simulink model "FA_18_Model_2016b"  (R2018a)
settings: Solver=ode45  StartTime=0.0  StopTime=700  FixedStep=0.1  MaxStep=0.1  RelTol=1e-3
PreLoadFcn:
  | load('FA_18_Parameters.mat')
undefined symbols (not defined in the file or in its folder): Earth, WGS84
libraries: aerolibfltsims x1, aerolibtransform2 x1, aerolibconvert2 x1
settings Model: Creator=User  LastModifiedBy=User
settings CodeAppCC: StateflowObjectComments=on

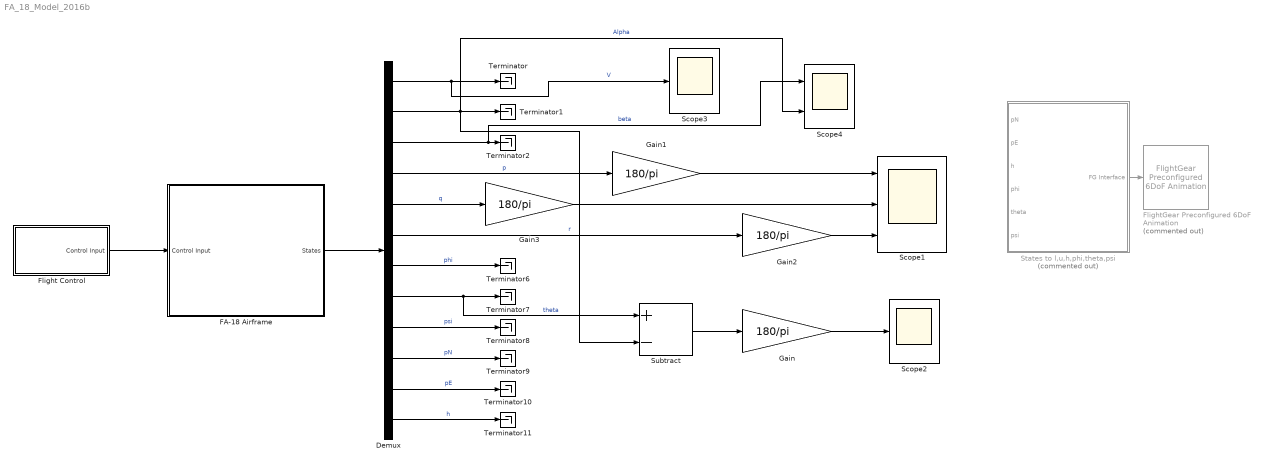
== system FA_18_Model_2016b ==
  Demux : Demux  Outputs=12
  FA-18 Airframe : Subsystem
  Flight Control : Subsystem
  FlightGear Preconfigured 6DoF Animation : aerolibfltsims/FlightGear Preconfigured 6DoF Animation  Commented=on  xFlightGearVersion=v2017.3  DestinationIpAddress=127.0.0.1  DestinationPort=5502  SampleTime=1/30
      settings: SourceProductName=Aerospace Blockset
  Gain{,1..3} (4 alike) : Gain  Gain=180/pi
  Scope1 : Scope  NumInputPorts=3
  Scope2 : Scope
  Scope3 : Scope
  Scope4 : Scope  NumInputPorts=2
  States to l,u,h,phi,theta,psi : Subsystem  Commented=on
  Subtract : Sum  Inputs=+-
  Terminator{,1..2,6..11} (9 alike) : Terminator
  wires:
  States to l,u,h,phi,theta,psi/1(FG Interface) -> FlightGear Preconfigured 6DoF Animation/1
  Flight Control/1(Control Input) -> FA-18 Airframe/1(Control Input)
  Demux/3 -> Scope4/1, Terminator2/1  "beta"
  Demux/2 -> Terminator1/1, Subtract/2, Scope4/2  "Alpha"
  Demux/8 -> Terminator7/1, Subtract/1  "theta"
  Demux/1 -> Scope3/1, Terminator/1  "V"
  Demux/7 -> Terminator6/1  "phi"
  Demux/4 -> Gain1/1  "p"
  Demux/10 -> Terminator9/1  "pN"
  Demux/9 -> Terminator8/1  "psi"
  FA-18 Airframe/1(States) -> Demux/1
  Demux/11 -> Terminator10/1  "pE"
  Demux/6 -> Gain2/1  "r"
  Demux/12 -> Terminator11/1  "h"
  Subtract/1 -> Gain/1
  Gain/1 -> Scope2/1
  Demux/5 -> Gain3/1  "q"
  Gain1/1 -> Scope1/1
  Gain2/1 -> Scope1/3
  Gain3/1 -> Scope1/2

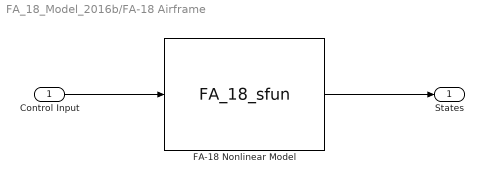
== system FA_18_Model_2016b/FA-18 Airframe ==
  Control Input : Inport
  FA-18 Nonlinear Model : S-Function  FunctionName=FA_18_sfun  Parameters=x0  SFunctionDeploymentMode=off  EnableBusSupport=off
  States : Outport
  wires:
  Control Input/1 -> FA-18 Nonlinear Model/1
  FA-18 Nonlinear Model/1 -> States/1

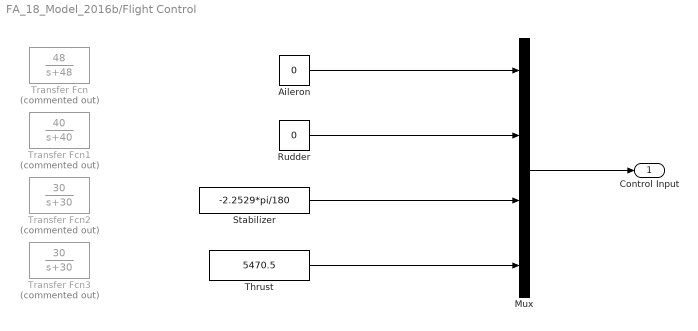
== system FA_18_Model_2016b/Flight Control ==
  Aileron : Constant  Value=0
  Mux : Mux
  Rudder : Constant  Value=0
  Stabilizer : Constant  Value=-2.2529*pi/180
  Thrust : Constant  Value=5470.5
  Transfer Fcn : TransferFcn  Commented=on  Numerator=48  Denominator=[1 48]
  Transfer Fcn1 : TransferFcn  Commented=on  Numerator=[40]  Denominator=[1 40]
  Transfer Fcn2 : TransferFcn  Commented=on  Numerator=[30]  Denominator=[1 30]
  Transfer Fcn3 : TransferFcn  Commented=on  Numerator=[30]  Denominator=[1 30]
  Control Input : Outport
  wires:
  Rudder/1 -> Mux/2
  Thrust/1 -> Mux/4
  Mux/1 -> Control Input/1
  Stabilizer/1 -> Mux/3
  Aileron/1 -> Mux/1

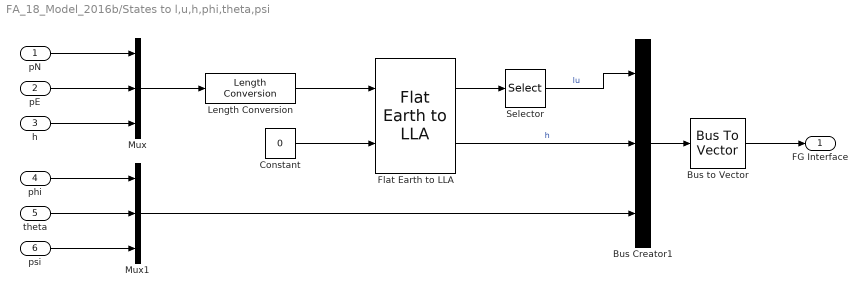
== system FA_18_Model_2016b/States to l,u,h,phi,theta,psi ==
  pN : Inport
  pE : Inport  Port=2
  h : Inport  Port=3
  phi : Inport  Port=4
  theta : Inport  Port=5
  psi : Inport  Port=6
  Bus Creator1 : BusCreator  Inputs=3
  Bus to Vector : BusToVector
  Constant : Constant  Value=0
  Flat Earth to LLA : aerolibtransform2/Flat Earth to LLA  units=Metric (MKS)  ptype=Earth (WGS84)  F=1/298.257223563  R=6378137  LL0=[50.1018 14.2632]  psi=0
  Length Conversion : aerolibconvert2/Length Conversion  IU=ft  OU=m
  Mux : Mux  Inputs=3
  Mux1 : Mux  Inputs=3
  Selector : Selector  IndexMode=Zero-based  InputPortWidth=2  IndexOptions=Index vector (dialog)  Indices=[1 0]  OutputSizes=1
  FG Interface : Outport
  wires:
  Constant/1 -> Flat Earth to LLA/2
  Length Conversion/1 -> Flat Earth to LLA/1
  Bus to Vector/1 -> FG Interface/1
  Bus Creator1/1 -> Bus to Vector/1
  Flat Earth to LLA/1 -> Selector/1
  Selector/1 -> Bus Creator1/1  "lu"
  Flat Earth to LLA/2 -> Bus Creator1/2  "h"
  pN/1 -> Mux/1
  pE/1 -> Mux/2
  h/1 -> Mux/3
  Mux/1 -> Length Conversion/1
  theta/1 -> Mux1/2
  phi/1 -> Mux1/1
  psi/1 -> Mux1/3
  Mux1/1 -> Bus Creator1/3
